simulink model "main"  (R2021a)
settings: Solver=ode113  StartTime=0.0  StopTime=100  RelTol=1e-13  AbsTol=1e-14
undefined symbols (not defined in the file or in its folder): Earth, initCond, Sensors, Spacecraft
libraries: aerolibutil x48, vrlib x31, dspsrcs4 x29, simulink x10, SADlibrary x8, commfilt2 x3, sharedtransform x3, dspfdesign x3, sharedutil x2, sharedTrackingLibrary x2, dspmathops x1
(part 1 of 3)
settings Model: Creator=matteo  LastModifiedBy=matteo
settings SolverCC: ZeroCrossControl=EnableAll  ZeroCrossAlgorithm=Adaptive  AlgebraicLoopSolver=TrustRegion  DecoupledContinuousIntegration=on
settings DebuggingCC: ReadBeforeWriteMsg=DisableAll  WriteAfterWriteMsg=DisableAll  WriteAfterReadMsg=DisableAll  MultiTaskDSMMsg=none  SFMachineParentedDataDiag=warning
settings ModelReferenceCC: UpdateModelReferenceTargets=IfOutOfDate
settings SFSimCC: SFSimEcho=off
settings SimscapeCC: SimscapeNormalizeSystem=off

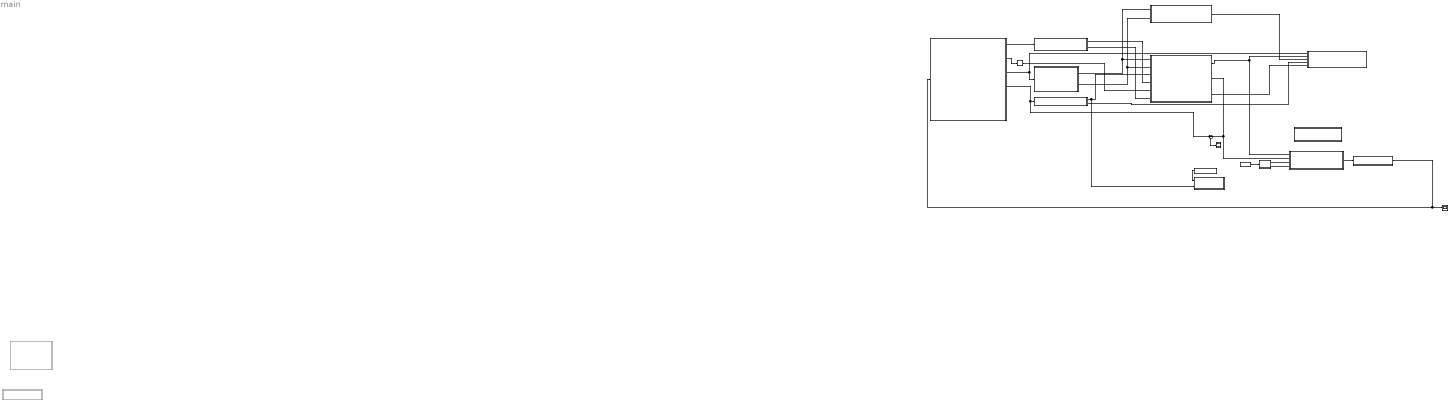
== system main ==
  Chart : Stateflow chart  Commented=on  TreatAsAtomicUnit=on
  Comparison : Subsystem
  Constant : Constant  Value=Spacecraft.str.inertia
  Control allocator : Subsystem
  Digital Clock : DigitalClock  SampleTime=1/1000
  Gyro reading : Subsystem
  Ideal control law : Subsystem
  Indipendent thrusters : Subsystem  Commented=on
  MATLAB Function : MATLAB Function  TreatAsAtomicUnit=on
  MATLAB Function4 : MATLAB Function  TreatAsAtomicUnit=on
  MPC : Subsystem
  Real physics : Subsystem
  Scope : Scope
  Scope4 : Scope
  Solve Whabba's problem : Subsystem
  Star sensor : Subsystem
  State estimator : Subsystem
  Subsystem1 : Subsystem
  Sum : Sum  Inputs=+-
  Zero-Order Hold : ZeroOrderHold  SampleTime=Sensors.sunSensor.freq
  wires:
  Real physics/4(Angular velocity [BF][rad/s]) -> Sum/1, Gyro reading/1(True ω [body refrence frame][rad/s])
  Real physics/2(Sun direction [NF]) -> Zero-Order Hold/1
  Real physics/1(Sun direction [BF]) -> Subsystem1/1(True Sun position [body reference frame][km])
  Real physics/3(q_B/N) -> Star sensor/1(Body attitude [Earth inertial frame]), Comparison/1(True attitude [ECI])
  Star sensor/1(Star 1 [SF]) -> Solve Whabba's problem/1(Stars [SF]), State estimator/1(Stars angles [sensor screen])
  Star sensor/2(in2) -> State estimator/2(MeasurementFcn1Inputs), Solve Whabba's problem/2(in2)
  Gyro reading/1(Measured ω [body reference frame][rad/s]) -> MATLAB Function4/2(omegaBody), State estimator/3(Gyro angular velocity [body frame])
  State estimator/1(Body frame attitude [ECI]) -> Comparison/2(Attitude Kalman [ECI]), Ideal control law/1(Body attitude [ECI])
  Solve Whabba's problem/1(Attitude quaternion) -> Comparison/3(Attitude Whabba's [ECI])
  State estimator/2(Angular velocity [body frame]) -> Sum/2, Ideal control law/2(Body angular speed [body frame])
  Gyro reading/2(Bias gyro true [body frame]) -> Comparison/4(Bias gyro true [body frame])
  State estimator/3(Gyro bias [body frame]) -> Comparison/5(Bias gyro Kalman [body frame])
  Sum/1 -> Scope/1
  MATLAB Function/1(q) -> Ideal control law/3(Reference attitude [ECI])
  MATLAB Function/2(omega) -> Ideal control law/4(Reference angular speed [ECI])
  Digital Clock/1 -> MATLAB Function/1(t)
  Control allocator/1(Real torque [body frame]) -> Real physics/1(Thrusters torque [BF][N m]), Scope4/1
  Subsystem1/1(Sun angles position [sensor axis]) -> State estimator/4(Sun sensor angles [SF])
  Zero-Order Hold/1 -> State estimator/5(Sun direction [NF])
  Subsystem1/2(Sensor attitude [body frame]) -> State estimator/6(Sun sensor attitude [BF])
  Constant/1 -> MATLAB Function4/1(J)
  Ideal control law/1(Ideal control torque [body frame]) -> Control allocator/1(Ideal torque [body frame])

== system main/Comparison ==
  True attitude [ECI] : Inport
  Attitude Kalman [ECI] : Inport  Port=2
  Attitude Whabba's [ECI] : Inport  Port=3
  Bias gyro true [body frame] : Inport  Port=4
  Bias gyro Kalman [body frame] : Inport  Port=5
  MATLAB Function : MATLAB Function  TreatAsAtomicUnit=on
  MATLAB Function1 : MATLAB Function  TreatAsAtomicUnit=on
  Quaternion Division1 : aerolibutil/Quaternion Division
      settings: SourceProductBaseCode=AE
  Quaternion Division2 : aerolibutil/Quaternion Division
      settings: SourceProductBaseCode=AE
  Scope : Scope  NumInputPorts=2
  Scope1 : Scope  NumInputPorts=2
  wires:
  True attitude [ECI]/1 -> Quaternion Division1/1, Quaternion Division2/1
  Attitude Kalman [ECI]/1 -> Quaternion Division2/2
  Attitude Whabba's [ECI]/1 -> Quaternion Division1/2
  Quaternion Division2/1 -> MATLAB Function1/1(q)  "UKF error"
  Bias gyro true [body frame]/1 -> Scope1/1
  Bias gyro Kalman [body frame]/1 -> Scope1/2
  MATLAB Function1/1(e) -> Scope/1  "UKF error"
  MATLAB Function/1(e) -> Scope/2  "Whabba's error"
  Quaternion Division1/1 -> MATLAB Function/1(q)  "Whabba's error"

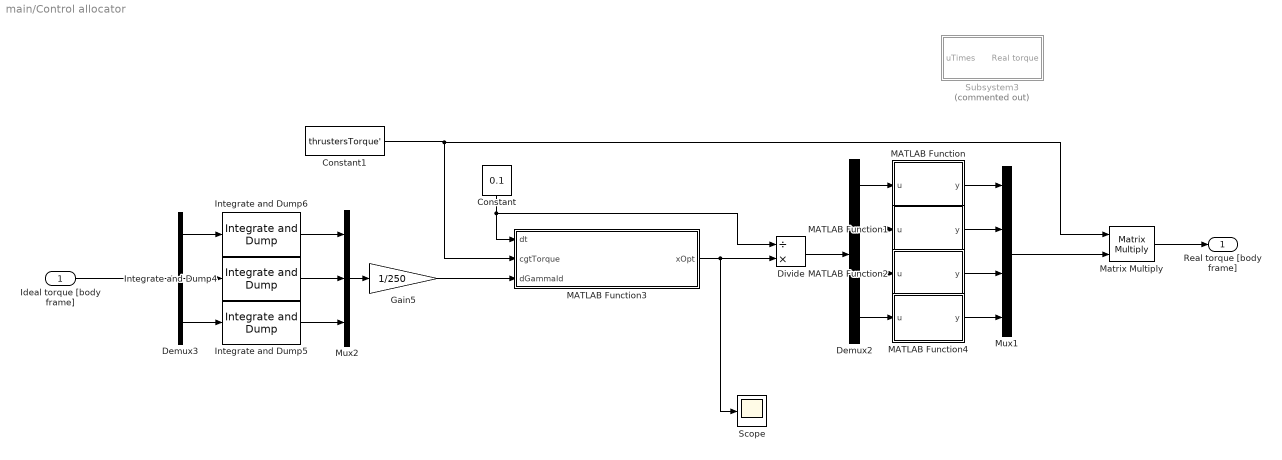
== system main/Control allocator ==
  Ideal torque [body frame] : Inport
  Constant : Constant  Value=0.1
  Constant1 : Constant  Value=thrustersTorque'  VectorParams1D=off
  Demux2 : Demux
  Demux3 : Demux  Outputs=3
  Divide : Product  Inputs=/*
  Gain5 : Gain  Gain=1/250
  Integrate and Dump4 : commfilt2/Integrate and Dump  obssamples=25  offsetsamples=0  nodump=off  roundingMode=Floor  overflowMode=off  outputDataTypeStr=Inherit: Same as accumulator  outputLastDataTypeStr=Inherit: Same as accumulator
  Integrate and Dump5 : commfilt2/Integrate and Dump  obssamples=25  offsetsamples=0  nodump=off  roundingMode=Floor  overflowMode=off  outputDataTypeStr=Inherit: Same as accumulator  outputLastDataTypeStr=Inherit: Same as accumulator
  Integrate and Dump6 : commfilt2/Integrate and Dump  obssamples=25  offsetsamples=0  nodump=off  roundingMode=Floor  overflowMode=off  outputDataTypeStr=Inherit: Same as accumulator  outputLastDataTypeStr=Inherit: Same as accumulator
  MATLAB Function : MATLAB Function  TreatAsAtomicUnit=on
  MATLAB Function1 : MATLAB Function  TreatAsAtomicUnit=on
  MATLAB Function2 : MATLAB Function  TreatAsAtomicUnit=on
  MATLAB Function3 : MATLAB Function  TreatAsAtomicUnit=on
  MATLAB Function4 : MATLAB Function  TreatAsAtomicUnit=on
  Matrix Multiply : Product  Multiplication=Matrix(*)
  Mux1 : Mux
  Mux2 : Mux  Inputs=3
  Scope : Scope
  Subsystem3 : Subsystem  Commented=on
  Real torque [body frame] : Outport
  wires:
  Integrate and Dump6/1 -> Mux2/1
  Demux3/2 -> Integrate and Dump4/1
  Gain5/1 -> MATLAB Function3/3(dGammaId)
  MATLAB Function3/1(xOpt) -> Divide/2, Scope/1
  Demux3/1 -> Integrate and Dump6/1
  Demux3/3 -> Integrate and Dump5/1
  Mux2/1 -> Gain5/1
  Integrate and Dump4/1 -> Mux2/2
  Ideal torque [body frame]/1 -> Demux3/1
  Integrate and Dump5/1 -> Mux2/3
  Constant/1 -> Divide/1, MATLAB Function3/1(dt)
  Demux2/4 -> MATLAB Function4/1(u)
  Mux1/1 -> Matrix Multiply/2
  MATLAB Function4/1(y) -> Mux1/4
  Matrix Multiply/1 -> Real torque [body frame]/1
  Demux2/3 -> MATLAB Function2/1(u)
  MATLAB Function/1(y) -> Mux1/1
  Demux2/1 -> MATLAB Function/1(u)
  MATLAB Function2/1(y) -> Mux1/3
  Constant1/1 -> MATLAB Function3/2(cgtTorque), Matrix Multiply/1
  Divide/1 -> Demux2/1
  MATLAB Function1/1(y) -> Mux1/2
  Demux2/2 -> MATLAB Function1/1(u)

== system main/Gyro reading ==
  True ω [body refrence frame][rad/s] : Inport
  Constant : Constant  Value=1e-3*randn(3,1)
  Cumulative Sum : dspmathops/Cumulative Sum  dim=Channels (running sum)  reset_popup=None  roundingMode=Floor  overflowMode=off  outputDataTypeStr=Inherit: Same as accumulator  outputMin=[]  outputMax=[]  outputLastDataTypeStr=Inherit: Same as accumulator
  Gain : Gain  Gain=sqrt(1/Sensors.gyro.freq)
  Random Source : dspsrcs4/Random Source  SrcType=Gaussian  NormMethod=Ziggurat  CltLength=12  MinVal=0  MaxVal=1  MeanVal=0  VarVal=Sensors.gyro.acc  RepMode=Not repeatable  rawSeed=1  IsInherit=off  SampMode=Discrete  SampTime=1/Sensors.gyro.freq  SampFrame=3  DataType=Double  OutComplex=Real  OutputFrames=off
  Random Source1 : dspsrcs4/Random Source  SrcType=Gaussian  NormMethod=Ziggurat  CltLength=12  MinVal=0  MaxVal=1  MeanVal=0  VarVal=Sensors.gyro.biasInstability  RepMode=Not repeatable  rawSeed=1  IsInherit=off  SampMode=Discrete  SampTime=1/Sensors.gyro.freq  SampFrame=3  DataType=Double  OutComplex=Real  OutputFrames=off
  Sum : Sum  Inputs=|++
  Sum1 : Sum  Inputs=|++
  Sum2 : Sum  Inputs=|++
  Zero-Order Hold : ZeroOrderHold  SampleTime=1/Sensors.gyro.freq
  Measured ω [body reference frame][rad/s] : Outport
  Bias gyro true [body frame] : Outport  Port=2
  wires:
  Sum2/1 -> Measured ω [body reference frame][rad/s]/1
  True ω [body refrence frame][rad/s]/1 -> Zero-Order Hold/1
  Cumulative Sum/1 -> Sum1/2
  Gain/1 -> Cumulative Sum/1
  Random Source1/1 -> Gain/1
  Constant/1 -> Sum1/1
  Zero-Order Hold/1 -> Sum/1
  Random Source/1 -> Sum/2
  Sum/1 -> Sum2/1
  Sum1/1 -> Bias gyro true [body frame]/1, Sum2/2

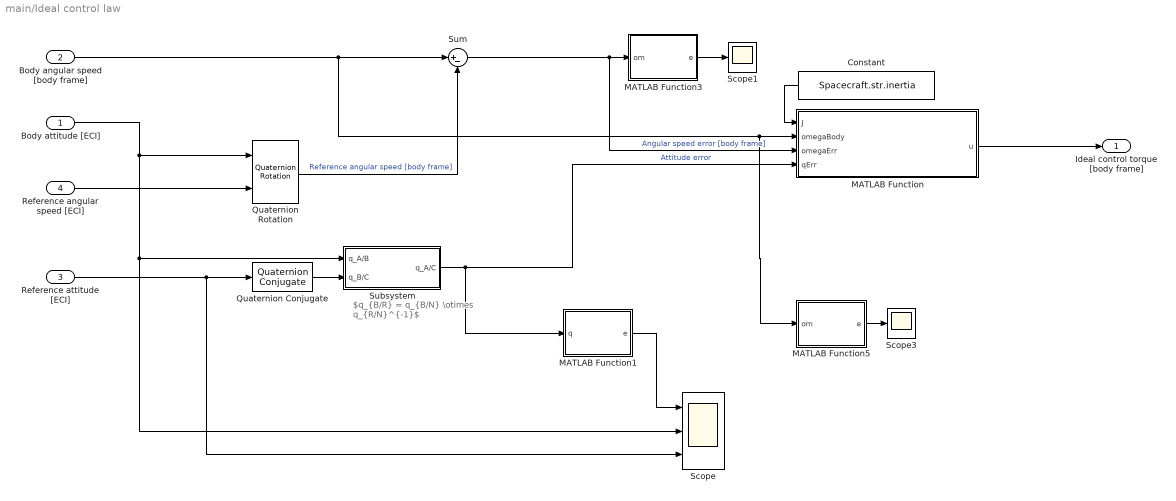
== system main/Ideal control law ==
  note: $q_{B/R} = q_{B/N} \otimes q_{R/N}^{-1}$
  Body attitude [ECI] : Inport
  Body angular speed [body frame] : Inport  Port=2
  Reference attitude [ECI] : Inport  Port=3
  Reference angular speed [ECI] : Inport  Port=4
  Constant : Constant  Value=Spacecraft.str.inertia
  MATLAB Function : MATLAB Function  TreatAsAtomicUnit=on
  MATLAB Function1 : MATLAB Function  TreatAsAtomicUnit=on
  MATLAB Function3 : MATLAB Function  TreatAsAtomicUnit=on
  MATLAB Function5 : MATLAB Function  TreatAsAtomicUnit=on
  Quaternion Conjugate : aerolibutil/Quaternion Conjugate
      settings: SourceProductBaseCode=AE
  Quaternion Rotation : aerolibutil/Quaternion Rotation
  Scope : Scope  NumInputPorts=3
  Scope1 : Scope
  Scope3 : Scope
  Subsystem : Subsystem
  Sum : Sum  Inputs=|+-
  Ideal control torque [body frame] : Outport
  wires:
  Subsystem/1(q_A/C) -> MATLAB Function/4(qErr), MATLAB Function1/1(q)  "Attitude error"
  Reference angular speed [ECI]/1 -> Quaternion Rotation/2
  Quaternion Rotation/1 -> Sum/2  "Reference angular speed [body frame]"
  Body angular speed [body frame]/1 -> MATLAB Function5/1(om), MATLAB Function/2(omegaBody), Sum/1
  Sum/1 -> MATLAB Function3/1(om), MATLAB Function/3(omegaErr)  "Angular speed error [body frame]"
  Constant/1 -> MATLAB Function/1(J)
  Reference attitude [ECI]/1 -> Scope/3, Quaternion Conjugate/1
  Body attitude [ECI]/1 -> Scope/2, Subsystem/1(q_A/B), Quaternion Rotation/1
  MATLAB Function1/1(e) -> Scope/1
  MATLAB Function3/1(e) -> Scope1/1
  MATLAB Function5/1(e) -> Scope3/1
  MATLAB Function/1(u) -> Ideal control torque [body frame]/1
  Quaternion Conjugate/1 -> Subsystem/2(q_B/C)

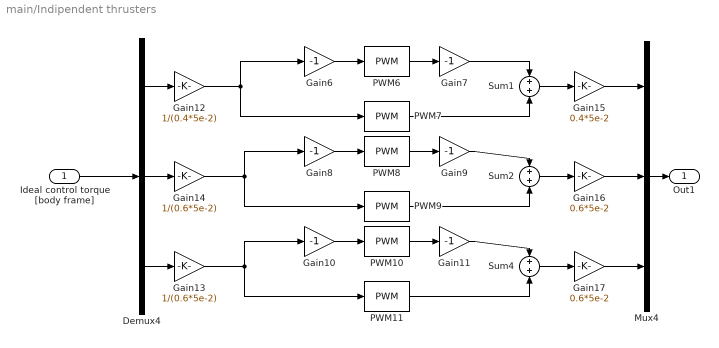
== system main/Indipendent thrusters ==
  Ideal control torque [body frame] : Inport
  Demux4 : Demux  Outputs=3
  Gain{6..11} (6 alike) : Gain  Gain=-1
  Gain12 : Gain  Gain=1/(0.4*5e-2)
  Gain13 : Gain  Gain=1/(0.6*5e-2)
  Gain14 : Gain  Gain=1/(0.6*5e-2)
  Gain15 : Gain  Gain=0.4*5e-2
  Gain16 : Gain  Gain=0.6*5e-2
  Gain17 : Gain  Gain=0.6*5e-2
  Mux4 : Mux  Inputs=3
  PWM{6..11} (6 alike) : simulink/Discontinuities/PWM  DisableCoverage=on  Period=0.5  DisallowZeroDutyCycle=off  RunAtFixedTimeIntervals=on  SampleTime=1/Sensors.gyroSamplingFreq
  Sum1 : Sum
  Sum2 : Sum
  Sum4 : Sum
  Out1 : Outport
  wires:
  PWM8/1 -> Gain9/1
  Mux4/1 -> Out1/1
  PWM11/1 -> Sum4/2
  Gain11/1 -> Sum4/1
  PWM6/1 -> Gain7/1
  Sum2/1 -> Gain16/1
  PWM10/1 -> Gain11/1
  Gain12/1 -> PWM7/1, Gain6/1
  Gain17/1 -> Mux4/3
  PWM7/1 -> Sum1/2
  Gain6/1 -> PWM6/1
  Gain16/1 -> Mux4/2
  Gain9/1 -> Sum2/1
  Gain14/1 -> PWM9/1, Gain8/1
  Demux4/1 -> Gain12/1
  Gain10/1 -> PWM10/1
  Gain13/1 -> PWM11/1, Gain10/1
  Demux4/2 -> Gain14/1
  Sum4/1 -> Gain17/1
  Ideal control torque [body frame]/1 -> Demux4/1
  Sum1/1 -> Gain15/1
  Gain8/1 -> PWM8/1
  Gain15/1 -> Mux4/1
  Demux4/3 -> Gain13/1
  PWM9/1 -> Sum2/2
  Gain7/1 -> Sum1/1

== system main/MPC ==
  Body attitude [ECI] : Inport
  Body angular speed [BF] : Inport  Port=2
  MATLAB Function : MATLAB Function  TreatAsAtomicUnit=on
  Ideal control law [BF] : Outport

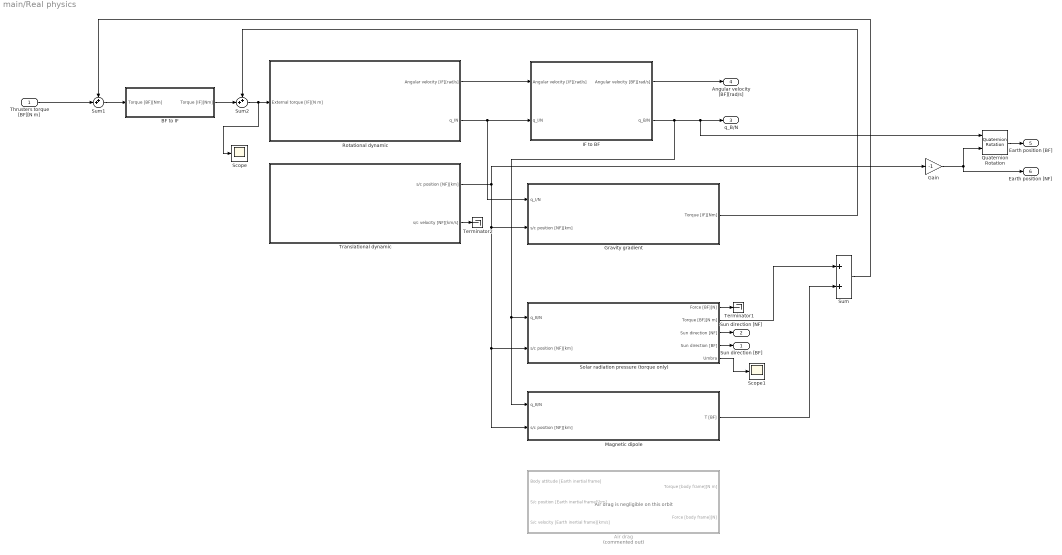
== system main/Real physics ==
  note: Air drag is negligible on this orbit
  Thrusters torque [BF][N m] : Inport  Unit=N*m
  Air drag : Subsystem  Commented=on
  BF to IF : Subsystem
  Gain : Gain  Gain=-1
  Gravity gradient : Subsystem
  IF to BF : Subsystem
  Magnetic dipole : Subsystem
  Quaternion Rotation : aerolibutil/Quaternion Rotation
  Rotational dynamic : Subsystem
  Scope : Scope
  Scope1 : Scope
  Solar radiation pressure (torque only) : Subsystem
  Sum : Sum
  Sum1 : Sum  Inputs=++|
  Sum2 : Sum  Inputs=++|
  Terminator1 : Terminator
  Terminator2 : Terminator
  Translational dynamic : Subsystem
  Sun direction [BF] : Outport  OutDataTypeStr=double  Unit=km
  Sun direction [NF] : Outport  Port=2
  q_B/N : Outport  Port=3
  Angular velocity [BF][rad/s] : Outport  Port=4
  Earth position [BF] : Outport  Port=5
  Earth position [NF] : Outport  Port=6
  wires:
  Sum/1 -> Sum1/1
  Solar radiation pressure (torque only)/1(Force [BF][N]) -> Terminator1/1
  Solar radiation pressure (torque only)/2(Torque [BF][N m]) -> Sum/1
  Thrusters torque [BF][N m]/1 -> Sum1/2
  Sum1/1 -> BF to IF/1(Torque [BF][Nm])
  Translational dynamic/1(s/c position [NF][km]) -> Solar radiation pressure (torque only)/2(s/c position [NF][km]), Magnetic dipole/2(s/c position [NF][km]), Gravity gradient/2(s/c position [NF][km]), Gain/1
  Rotational dynamic/1(Angular velocity [IF][rad/s]) -> IF to BF/1(Angular velocity [IF][rad/s])
  IF to BF/1(Angular velocity [BF][rad/s]) -> Angular velocity [BF][rad/s]/1
  IF to BF/2(q_B/N) -> Magnetic dipole/1(q_B/N), Solar radiation pressure (torque only)/1(q_B/N), q_B/N/1, Quaternion Rotation/1
  Solar radiation pressure (torque only)/3(Sun direction [NF]) -> Sun direction [NF]/1
  Solar radiation pressure (torque only)/4(Sun direction [BF]) -> Sun direction [BF]/1
  Solar radiation pressure (torque only)/5(Umbra) -> Scope1/1
  BF to IF/1(Torque [IF][Nm]) -> Sum2/2
  Sum2/1 -> Scope/1, Rotational dynamic/1(External torque [IF][N m])
  Translational dynamic/2(s/c velocity [NF][km/s]) -> Terminator2/1
  Gravity gradient/1(Torque [IF][Nm]) -> Sum2/1
  Rotational dynamic/2(q_IN) -> Gravity gradient/1(q_I/N), IF to BF/2(q_I/N)
  Gain/1 -> Earth position [NF]/1, Quaternion Rotation/2
  Quaternion Rotation/1 -> Earth position [BF]/1
  Magnetic dipole/1(T [BF]) -> Sum/2

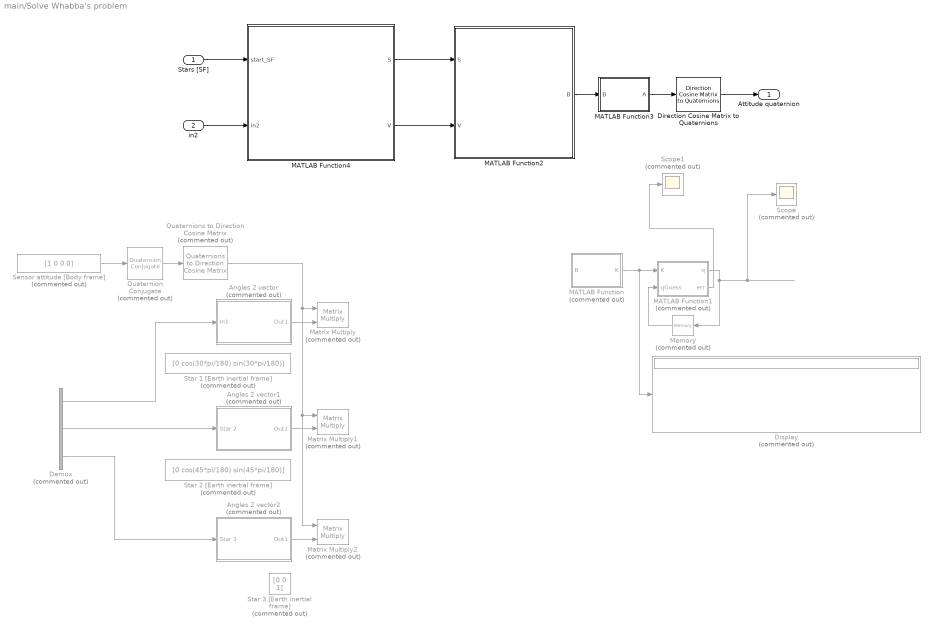
== system main/Solve Whabba's problem ==
  Stars [SF] : Inport
  in2 : Inport  Port=2
  Angles 2 vector : Subsystem  Commented=on
  Angles 2 vector1 : Subsystem  Commented=on
  Angles 2 vector2 : Subsystem  Commented=on
  Demux : Demux  Commented=on  Outputs=3
  Direction Cosine Matrix to Quaternions : sharedtransform/Direction Cosine Matrix  to Quaternions  aMode=0  action=None  tolerance=eps(2)
      settings: SourceProductBaseCode=AE,PW,DR,MT,UV,VE
  Display : Display  Commented=on
  MATLAB Function : MATLAB Function  Commented=on  TreatAsAtomicUnit=on
  MATLAB Function1 : MATLAB Function  Commented=on  TreatAsAtomicUnit=on
  MATLAB Function2 : MATLAB Function  TreatAsAtomicUnit=on
  MATLAB Function3 : MATLAB Function  TreatAsAtomicUnit=on
  MATLAB Function4 : MATLAB Function  TreatAsAtomicUnit=on
  Matrix Multiply : Product  Commented=on  Multiplication=Matrix(*)
  Matrix Multiply1 : Product  Commented=on  Multiplication=Matrix(*)
  Matrix Multiply2 : Product  Commented=on  Multiplication=Matrix(*)
  Memory : Memory  Commented=on  InitialCondition=[1 0 0 0]
  Quaternion Conjugate : aerolibutil/Quaternion Conjugate  Commented=on
      settings: SourceProductBaseCode=AE
  Quaternions to Direction Cosine Matrix : sharedtransform/Quaternions to  Direction Cosine Matrix  Commented=on  aMode=aMode
      settings: SourceProductBaseCode=AE,PW,DR,MT,UV,VE
  Scope : Scope  Commented=on
  Scope1 : Scope  Commented=on
  Sensor attitude [Body frame] : Constant  Commented=on  Value=[1 0 0 0]
  Star 1 [Earth inertial frame] : Constant  Commented=on  Value=[0 cos(30*pi/180) sin(30*pi/180)]
  Star 2 [Earth inertial frame] : Constant  Commented=on  Value=[0 cos(45*pi/180) sin(45*pi/180)]
  Star 3 [Earth inertial frame] : Constant  Commented=on  Value=[0 0 1]
  Attitude quaternion : Outport
  wires:
  Demux/1 -> Angles 2 vector/1(In1)
  Demux/2 -> Angles 2 vector1/1(Star 2)
  Demux/3 -> Angles 2 vector2/1(Star 3)
  Angles 2 vector/1(Out1) -> Matrix Multiply/2
  MATLAB Function2/1(B) -> MATLAB Function3/1(B)
  MATLAB Function/1(K) -> Display/1, MATLAB Function1/1(K)
  MATLAB Function1/1(q) -> Memory/1, Scope/1
  Sensor attitude [Body frame]/1 -> Quaternion Conjugate/1
  Quaternion Conjugate/1 -> Quaternions to Direction Cosine Matrix/1
  Quaternions to Direction Cosine Matrix/1 -> Matrix Multiply2/1, Matrix Multiply1/1, Matrix Multiply/1
  Angles 2 vector2/1(Out1) -> Matrix Multiply2/2
  Angles 2 vector1/1(Out1) -> Matrix Multiply1/2
  Memory/1 -> MATLAB Function1/2(qGuess)
  MATLAB Function1/2(err) -> Scope1/1
  MATLAB Function3/1(A) -> Direction Cosine Matrix to Quaternions/1
  Direction Cosine Matrix to Quaternions/1 -> Attitude quaternion/1
  MATLAB Function4/1(S) -> MATLAB Function2/1(S)
  MATLAB Function4/2(V) -> MATLAB Function2/2(V)
  Stars [SF]/1 -> MATLAB Function4/1(start_SF)
  in2/1 -> MATLAB Function4/2(in2)

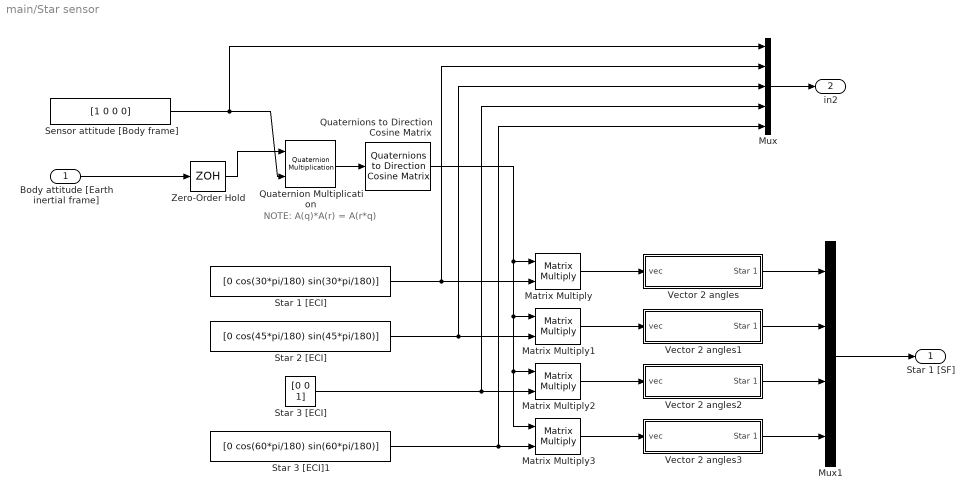
== system main/Star sensor ==
  note: NOTE: A(q)*A(r) = A(r*q)
  Body attitude [Earth inertial frame] : Inport
  Matrix Multiply{,1..3} (4 alike) : Product  Multiplication=Matrix(*)
  Mux : Mux  Inputs=5
  Mux1 : Mux
  Quaternion Multiplication : aerolibutil/Quaternion Multiplication
  Quaternions to Direction Cosine Matrix : sharedtransform/Quaternions to  Direction Cosine Matrix  aMode=aMode
      settings: SourceProductBaseCode=AE,PW,DR,MT,UV,VE
  Sensor attitude [Body frame] : Constant  Value=[1 0 0 0]
  Star 1 [ECI] : Constant  Value=[0 cos(30*pi/180) sin(30*pi/180)]
  Star 2 [ECI] : Constant  Value=[0 cos(45*pi/180) sin(45*pi/180)]
  Star 3 [ECI] : Constant  Value=[0 0 1]
  Star 3 [ECI]1 : Constant  Value=[0 cos(60*pi/180) sin(60*pi/180)]
  Vector 2 angles : Subsystem
  Vector 2 angles1 : Subsystem
  Vector 2 angles2 : Subsystem
  Vector 2 angles3 : Subsystem
  Zero-Order Hold : ZeroOrderHold  SampleTime=1/Sensors.starTracker.freq
  Star 1 [SF] : Outport
  in2 : Outport  Port=2
  wires:
  Body attitude [Earth inertial frame]/1 -> Zero-Order Hold/1
  Sensor attitude [Body frame]/1 -> Quaternion Multiplication/2, Mux/1
  Quaternion Multiplication/1 -> Quaternions to Direction Cosine Matrix/1
  Star 1 [ECI]/1 -> Matrix Multiply/2, Mux/2
  Star 2 [ECI]/1 -> Mux/3, Matrix Multiply1/2
  Star 3 [ECI]/1 -> Mux/4, Matrix Multiply2/2
  Quaternions to Direction Cosine Matrix/1 -> Matrix Multiply3/1, Matrix Multiply2/1, Matrix Multiply1/1, Matrix Multiply/1
  Matrix Multiply/1 -> Vector 2 angles/1(vec)
  Matrix Multiply2/1 -> Vector 2 angles2/1(vec)
  Matrix Multiply1/1 -> Vector 2 angles1/1(vec)
  Vector 2 angles1/1(Star 1) -> Mux1/2
  Vector 2 angles2/1(Star 1) -> Mux1/3
  Vector 2 angles/1(Star 1) -> Mux1/1
  Mux/1 -> in2/1
  Zero-Order Hold/1 -> Quaternion Multiplication/1
  Mux1/1 -> Star 1 [SF]/1
  Star 3 [ECI]1/1 -> Mux/5, Matrix Multiply3/2
  Matrix Multiply3/1 -> Vector 2 angles3/1(vec)
  Vector 2 angles3/1(Star 1) -> Mux1/4

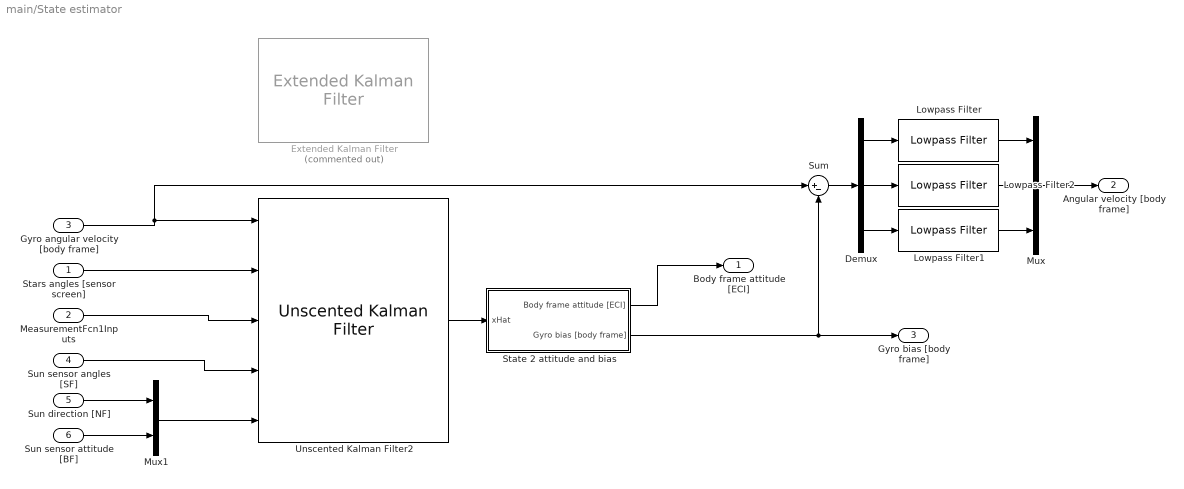
== system main/State estimator ==
  Stars angles [sensor screen] : Inport
  MeasurementFcn1Inputs : Inport  Port=2
  Gyro angular velocity [body frame] : Inport  Port=3
  Sun sensor angles [SF] : Inport  Port=4
  Sun direction [NF] : Inport  Port=5
  Sun sensor attitude [BF] : Inport  Port=6
  Demux : Demux  Outputs=3
  Extended Kalman Filter : sharedTrackingLibrary/Extended Kalman Filter  Commented=on  StateTransitionFcn=statePropagation  HasStateTransitionJacobianFcn=off  HasAdditiveProcessNoise=Nonadditive  ProcessNoise=diag([Sensors.gyro.acc* [1 1 1], Sensors.gyro.biasInstability* [1 1 1]])  HasTimeVaryingProcessNoise=off  HasStateTransitionFcnExtraArgument=1  InitialState=[Spacecraft.initialAttitude 0 0 0]'  InitialStateCovariance=1e-6*eye(7)  MeasurementFcn1=simulateStarTracker  HasMeasurementJacobianFcn1=off  HasMeasurementEnablePort1=off  HasAdditiveMeasurementNoise1=Additive  MeasurementNoise1=diag(repmat([Sensors.sunSensor.aboutBoresight Sensors.sunSensor.crossBoresight Sensors.sunSensor.crossBoresight],[1 4]));  HasTimeVaryingMeasurementNoise1=off  HasMeasurementFcnExtraArgument1=1  MeasurementFcn2=simulateSunSensor  HasMeasurementJacobianFcn2=off  HasMeasurementEnablePort2=off  HasAdditiveMeasurementNoise2=Additive  MeasurementNoise2=diag([Sensors.sunSensor.aboutBoresight Sensors.sunSensor.crossBoresight Sensors.sunSensor.crossBoresight]);  HasTimeVaryingMeasurementNoise2=off  HasMeasurementFcnExtraArgument2=1  MeasurementFcn3=myMeasurementFcn  HasMeasurementJacobianFcn3=off  HasMeasurementEnablePort3=off  HasAdditiveMeasurementNoise3=Additive  MeasurementNoise3=1  HasTimeVaryingMeasurementNoise3=off  HasMeasurementFcnExtraArgument3=0  MeasurementFcn4=myMeasurementFcn  HasMeasurementJacobianFcn4=off  HasMeasurementEnablePort4=off  HasAdditiveMeasurementNoise4=Additive  MeasurementNoise4=1  HasTimeVaryingMeasurementNoise4=off  HasMeasurementFcnExtraArgument4=0  MeasurementFcn5=myMeasurementFcn  HasMeasurementJacobianFcn5=off  HasMeasurementEnablePort5=off  HasAdditiveMeasurementNoise5=Additive  MeasurementNoise5=1  HasTimeVaryingMeasurementNoise5=off  HasMeasurementFcnExtraArgument5=0  EnableMultirate=on  StateTransitionFcnSampleTime=1/Sensors.gyro.freq  MeasurementFcn1SampleTime=1/Sensors.starTracker.freq  MeasurementFcn2SampleTime=1/Sensors.sunSensor.freq  MeasurementFcn3SampleTime=1  MeasurementFcn4SampleTime=1  MeasurementFcn5SampleTime=1  UseCurrentEstimator=on  OutputStateCovariance=off  DataType=double  SampleTime=1  NumberOfMeasurements=2
      settings: SourceProductBaseCode=CT,DR,TF,ID,LP,NV,AR,RO,RR,UV,VE
  Lowpass Filter : dspfdesign/Lowpass Filter  FilterType=FIR  DesignForMinimumOrder=on  FilterOrder=50  PassbandFrequency=20  StopbandFrequency=40  PassbandRipple=0.0001  StopbandAttenuation=80  InheritSampleRate=off  SampleRate=250  SimulateUsing=Interpreted execution  roundingMode=Floor  coeffsDataTypeStr=fixdt(1,16)
  Lowpass Filter1 : dspfdesign/Lowpass Filter  FilterType=FIR  DesignForMinimumOrder=on  FilterOrder=50  PassbandFrequency=20  StopbandFrequency=40  PassbandRipple=0.0001  StopbandAttenuation=80  InheritSampleRate=off  SampleRate=250  SimulateUsing=Interpreted execution  roundingMode=Floor  coeffsDataTypeStr=fixdt(1,16)
  Lowpass Filter2 : dspfdesign/Lowpass Filter  FilterType=FIR  DesignForMinimumOrder=on  FilterOrder=50  PassbandFrequency=20  StopbandFrequency=40  PassbandRipple=0.0001  StopbandAttenuation=80  InheritSampleRate=off  SampleRate=250  SimulateUsing=Interpreted execution  roundingMode=Floor  coeffsDataTypeStr=fixdt(1,16)
  Mux : Mux  Inputs=3
  Mux1 : Mux  Inputs=2
  State 2 attitude and bias : Subsystem
  Sum : Sum  Inputs=|+-
  Unscented Kalman Filter2 : sharedTrackingLibrary/Unscented Kalman Filter  StateTransitionFcn=statePropagation  HasAdditiveProcessNoise=Nonadditive  ProcessNoise=diag([Sensors.gyro.acc* [1 1 1], Sensors.gyro.biasInstability * [1 1 1]])  HasTimeVaryingProcessNoise=off  HasStateTransitionFcnExtraArgument=1  InitialState=[Spacecraft.initialAttitude 0 0 0]'  InitialStateCovariance=1e-6*eye(7)  Alpha=1e-3  Beta=2  Kappa=0  MeasurementFcn1=simulateStarTracker  HasMeasurementEnablePort1=off  HasAdditiveMeasurementNoise1=Nonadditive  MeasurementNoise1=diag(repmat([Sensors.starTracker.aboutBoresight Sensors.starTracker.crossBoresight],[1 4]));  HasTimeVaryingMeasurementNoise1=off  HasMeasurementFcnExtraArgument1=1  MeasurementFcn2=simulateSunSensor  HasMeasurementEnablePort2=off  HasAdditiveMeasurementNoise2=Nonadditive  MeasurementNoise2=diag([Sensors.sunSensor.aboutBoresight Sensors.sunSensor.crossBoresight]);  HasTimeVaryingMeasurementNoise2=off  HasMeasurementFcnExtraArgument2=1  MeasurementFcn3=simulateSunSensor  HasMeasurementEnablePort3=off  HasAdditiveMeasurementNoise3=Additive  MeasurementNoise3=(.1*pi/180)^2*eye(2)  HasTimeVaryingMeasurementNoise3=off  HasMeasurementFcnExtraArgument3=1  MeasurementFcn4=myMeasurementFcn  HasMeasurementEnablePort4=off  HasAdditiveMeasurementNoise4=Additive  MeasurementNoise4=1  HasTimeVaryingMeasurementNoise4=off  HasMeasurementFcnExtraArgument4=0  MeasurementFcn5=myMeasurementFcn  HasMeasurementEnablePort5=off  HasAdditiveMeasurementNoise5=Additive  MeasurementNoise5=1  HasTimeVaryingMeasurementNoise5=off  HasMeasurementFcnExtraArgument5=0  EnableMultirate=on  StateTransitionFcnSampleTime=1/Sensors.gyro.freq  MeasurementFcn1SampleTime=1/Sensors.starTracker.freq  MeasurementFcn2SampleTime=1/Sensors.sunSensor.freq  MeasurementFcn3SampleTime=Sensors.sunSensorSamplingFreq  MeasurementFcn4SampleTime=1  MeasurementFcn5SampleTime=1  UseCurrentEstimator=on  OutputStateCovariance=off  DataType=double  SampleTime=0.01  NumberOfMeasurements=2
      settings: SourceProductBaseCode=CT,DR,TF,ID,LP,NV,AR,RO,RR,UV,VE
  Body frame attitude [ECI] : Outport
  Angular velocity [body frame] : Outport  Port=2
  Gyro bias [body frame] : Outport  Port=3
  wires:
  MeasurementFcn1Inputs/1 -> Unscented Kalman Filter2/3
  State 2 attitude and bias/2(Gyro bias [body frame]) -> Sum/2, Gyro bias [body frame]/1
  State 2 attitude and bias/1(Body frame attitude [ECI]) -> Body frame attitude [ECI]/1
  Unscented Kalman Filter2/1 -> State 2 attitude and bias/1(xHat)
  Stars angles [sensor screen]/1 -> Unscented Kalman Filter2/2
  Demux/1 -> Lowpass Filter/1
  Demux/2 -> Lowpass Filter2/1
  Demux/3 -> Lowpass Filter1/1
  Lowpass Filter/1 -> Mux/1
  Lowpass Filter1/1 -> Mux/3
  Lowpass Filter2/1 -> Mux/2
  Sum/1 -> Demux/1
  Mux/1 -> Angular velocity [body frame]/1
  Gyro angular velocity [body frame]/1 -> Unscented Kalman Filter2/1, Sum/1
  Sun sensor angles [SF]/1 -> Unscented Kalman Filter2/4
  Mux1/1 -> Unscented Kalman Filter2/5
  Sun direction [NF]/1 -> Mux1/1
  Sun sensor attitude [BF]/1 -> Mux1/2

== system main/Subsystem1 ==
  True Sun position [body reference frame][km] : Inport
  MATLAB Function1 : MATLAB Function  TreatAsAtomicUnit=on
  Sensor orientation : Constant  Value=[1 0 0 0]
  Sensor orientation1 : Constant  Value=[cos(pi/4) 0 sin(pi/4) 0]
  Sensor orientation2 : Constant  Value=[cos(pi/2) 0 sin(pi/2) 0]
  Sensor orientation3 : Constant  Value=[cos(pi/4) 0 -sin(pi/4) 0]
  Sensor orientation4 : Constant  Value=[cos(pi/4) -sin(pi/4) 0 0]
  Sensor orientation5 : Constant  Value=[cos(pi/4) sin(pi/4) 0 0]
  Sun sensor reading : Subsystem
  Sun sensor reading1 : Subsystem
  Sun sensor reading2 : Subsystem
  Sun sensor reading3 : Subsystem
  Sun sensor reading4 : Subsystem
  Sun sensor reading5 : Subsystem
  Sun angles position [sensor axis] : Outport  PortDimensions=2
  Sensor attitude [body frame] : Outport  Port=2  PortDimensions=4
  wires:
  True Sun position [body reference frame][km]/1 -> Sun sensor reading2/1(True Sun position [body reference frame][km]), Sun sensor reading1/1(True Sun position [body reference frame][km]), Sun sensor reading/1(True Sun position [body reference frame][km]), Sun sensor reading3/1(True Sun position [body reference frame][km]), Sun sensor reading5/1(True Sun position [body reference frame][km]), Sun sensor reading4/1(True Sun position [body reference frame][km])
  MATLAB Function1/2(sensAtt) -> Sensor attitude [body frame]/1
  Sun sensor reading/1(Sun angles position [sensor axis]) -> MATLAB Function1/1(s1)
  MATLAB Function1/1(s) -> Sun angles position [sensor axis]/1
  Sensor orientation/1 -> MATLAB Function1/2(q_SB1), Sun sensor reading/2(q_S/B)
  Sun sensor reading1/1(Sun angles position [sensor axis]) -> MATLAB Function1/3(s2)
  Sun sensor reading2/1(Sun angles position [sensor axis]) -> MATLAB Function1/5(s3)
  Sun sensor reading3/1(Sun angles position [sensor axis]) -> MATLAB Function1/7(s4)
  Sun sensor reading4/1(Sun angles position [sensor axis]) -> MATLAB Function1/9(s5)
  Sun sensor reading5/1(Sun angles position [sensor axis]) -> MATLAB Function1/11(s6)
  Sensor orientation1/1 -> Sun sensor reading1/2(q_S/B), MATLAB Function1/4(q_SB2)
  Sensor orientation2/1 -> Sun sensor reading2/2(q_S/B), MATLAB Function1/6(q_SB3)
  Sensor orientation3/1 -> Sun sensor reading3/2(q_S/B), MATLAB Function1/8(q_SB4)
  Sensor orientation4/1 -> Sun sensor reading4/2(q_S/B), MATLAB Function1/10(q_SB5)
  Sensor orientation5/1 -> Sun sensor reading5/2(q_S/B), MATLAB Function1/12(q_SB6)

== system main/Control allocator/Subsystem3 ==
  uTimes : Inport
  Constant : Constant  Value=thrustersTorque'  VectorParams1D=off
  Demux1 : Demux  Commented=on
  Demux2 : Demux
  Gain : Gain  Gain=1/(50/500)
  MATLAB Function : MATLAB Function  TreatAsAtomicUnit=on
  MATLAB Function1 : MATLAB Function  TreatAsAtomicUnit=on
  MATLAB Function2 : MATLAB Function  TreatAsAtomicUnit=on
  MATLAB Function3 : MATLAB Function  TreatAsAtomicUnit=on
  Matrix Multiply : Product  Multiplication=Matrix(*)
  Mux1 : Mux  Commented=on
  Mux2 : Mux
  PWM{13,17..18,21} (4 alike) : simulink/Discontinuities/PWM  Commented=on  DisableCoverage=on  Period=0.1  DisallowZeroDutyCycle=off  RunAtFixedTimeIntervals=on  SampleTime=0.1
  Real torque : Outport
  wires:
  Mux2/1 -> Matrix Multiply/2
  Constant/1 -> Matrix Multiply/1
  Matrix Multiply/1 -> ?
  PWM18/1 -> Mux1/3
  PWM21/1 -> Mux1/1
  Demux1/2 -> PWM17/1
  PWM17/1 -> Mux1/2
  PWM13/1 -> Mux1/4
  Demux1/1 -> PWM21/1
  Demux1/4 -> PWM13/1
  Demux1/3 -> PWM18/1
  uTimes/1 -> ?
  Demux2/1 -> MATLAB Function/1(u)
  Gain/1 -> Demux2/1
  MATLAB Function/1(y) -> Mux2/1
  Demux2/2 -> MATLAB Function1/1(u)
  MATLAB Function1/1(y) -> Mux2/2
  Demux2/3 -> MATLAB Function2/1(u)
  MATLAB Function2/1(y) -> Mux2/3
  Demux2/4 -> MATLAB Function3/1(u)
  MATLAB Function3/1(y) -> Mux2/4

== system main/Ideal control law/Subsystem ==
  q_A/B : Inport
  q_B/C : Inport  Port=2
  Quaternion Multiplication : aerolibutil/Quaternion Multiplication
  q_A/C : Outport
  wires:
  q_A/B/1 -> Quaternion Multiplication/2
  q_B/C/1 -> Quaternion Multiplication/1
  Quaternion Multiplication/1 -> q_A/C/1

== system main/Real physics/Air drag ==
  Body attitude [Earth inertial frame] : Inport  Unit=1
  S/c position [Earth inertial frame][km] : Inport  Port=2  OutDataTypeStr=double  Unit=km  PortDimensions=3
  S/c velocity [Earth inertial frame][km/s] : Inport  Port=3  OutDataTypeStr=double  Unit=km/s
  Air density : Subsystem
  Constant : Constant  Value=Spacecraft  OutDataTypeStr=Bus: SpacecraftDT
  Constant1 : Constant  Value=Earth.equatorialRadius
  Constant2 : Constant  Value=2*pi/Earth.siderealDay
  Cross Product : vrlib/Utilities/Cross Product
  Gain : Gain  Gain=[0;0;1]
  MATLAB Function : MATLAB Function  TreatAsAtomicUnit=on
  Sum : Sum  Inputs=+-|
  Sum1 : Sum  Inputs=|-+
  Terminator : Terminator
  Vector magnitude and direction1 : SADlibrary/Vector magnitude and direction  SystemSampleTime=-1  VariantActivationTime=update diagram  Latency=0  AutoFrameSizeCalculation=off
  Vector rotate : SADlibrary/Vector rotate  SystemSampleTime=-1  VariantActivationTime=update diagram  Latency=0  AutoFrameSizeCalculation=off
  Torque [body frame][N m] : Outport  Unit=N*m
  Force [body frame][N] : Outport  Port=2  Unit=N
  wires:
  Vector magnitude and direction1/1 -> Sum/1
  Body attitude [Earth inertial frame]/1 -> Vector rotate/1
  MATLAB Function/2(T) -> Torque [body frame][N m]/1
  MATLAB Function/1(F) -> Force [body frame][N]/1
  Constant/1 -> MATLAB Function/3(Spacecraft)
  Vector rotate/1 -> MATLAB Function/2(relVel)
  Constant1/1 -> Sum/2
  Constant2/1 -> Gain/1
  Gain/1 -> Cross Product/1
  Cross Product/1 -> Sum1/1
  S/c velocity [Earth inertial frame][km/s]/1 -> Sum1/2
  Sum1/1 -> Vector rotate/2
  Sum/1 -> Air density/1(Height)
  Air density/1(Air density) -> MATLAB Function/1(rho)
  S/c position [Earth inertial frame][km]/1 -> Vector magnitude and direction1/1, Cross Product/2
  Vector magnitude and direction1/2 -> Terminator/1

== system main/Real physics/BF to IF ==
  Torque [BF][Nm] : Inport
  Constant : Constant  Value=Spacecraft.str.qIB
  Quaternion Rotation1 : aerolibutil/Quaternion Rotation
  Torque [IF][Nm] : Outport
  wires:
  Quaternion Rotation1/1 -> Torque [IF][Nm]/1
  Torque [BF][Nm]/1 -> Quaternion Rotation1/2
  Constant/1 -> Quaternion Rotation1/1

== system main/Real physics/Gravity gradient ==
  q_I/N : Inport
  s/c position [NF][km] : Inport  Port=2
  Constant : Constant  Value=Earth.mu
  Constant1 : Constant  Value=Spacecraft.str.inertia
  MATLAB Function : MATLAB Function  TreatAsAtomicUnit=on
  Quaternion Rotation : aerolibutil/Quaternion Rotation
  Torque [IF][Nm] : Outport
  wires:
  q_I/N/1 -> Quaternion Rotation/1
  s/c position [NF][km]/1 -> Quaternion Rotation/2
  MATLAB Function/1(torque_IF) -> Torque [IF][Nm]/1
  Constant/1 -> MATLAB Function/1(mu)
  Constant1/1 -> MATLAB Function/2(J)
  Quaternion Rotation/1 -> MATLAB Function/3(position_IF)

== system main/Real physics/IF to BF ==
  Angular velocity [IF][rad/s] : Inport
  q_I/N : Inport  Port=2
  Constant : Constant  Value=Spacecraft.str.qIB
  Quaternion Conjugate : aerolibutil/Quaternion Conjugate
      settings: SourceProductBaseCode=AE
  Quaternion Multiplication : aerolibutil/Quaternion Multiplication
  Quaternion Rotation1 : aerolibutil/Quaternion Rotation
  Angular velocity [BF][rad/s] : Outport
  q_B/N : Outport  Port=2
  wires:
  q_I/N/1 -> Quaternion Multiplication/1
  Quaternion Multiplication/1 -> q_B/N/1
  Constant/1 -> Quaternion Conjugate/1
  Quaternion Rotation1/1 -> Angular velocity [BF][rad/s]/1
  Angular velocity [IF][rad/s]/1 -> Quaternion Rotation1/2
  Quaternion Conjugate/1 -> Quaternion Multiplication/2, Quaternion Rotation1/1

== system main/Real physics/Magnetic dipole ==
  q_B/N : Inport
  s/c position [NF][km] : Inport  Port=2
  Constant : Constant  Value=Spacecraft.str.magDip
  Cross Product : vrlib/Utilities/Cross Product
  Subsystem2 : Subsystem
  T [BF] : Outport
  wires:
  Constant/1 -> Cross Product/1
  q_B/N/1 -> Subsystem2/1(q_A/B)
  s/c position [NF][km]/1 -> Subsystem2/2(r_NF)
  Subsystem2/1(B [BF]) -> Cross Product/2
  Cross Product/1 -> T [BF]/1

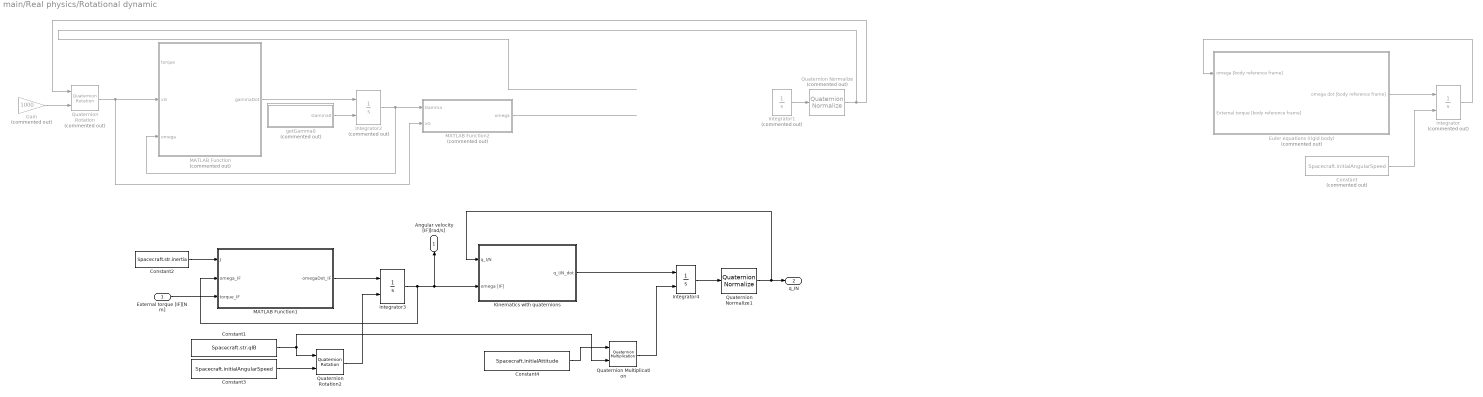
== system main/Real physics/Rotational dynamic ==
  External torque [IF][N m] : Inport
  Constant : Constant  Commented=on  Value=Spacecraft.initialAngularSpeed
  Constant1 : Constant  Value=Spacecraft.str.qIB
  Constant2 : Constant  Value=Spacecraft.str.inertia
  Constant3 : Constant  Value=Spacecraft.initialAngularSpeed
  Constant4 : Constant  Value=Spacecraft.initialAttitude
  "Euler equations (rigid body) " : Subsystem  Commented=on
  Gain : Gain  Commented=on  Gain=1000
  Integrator : Integrator  Commented=on  InitialConditionSource=external  InitialCondition=initCond
  Integrator1 : Integrator  Commented=on  InitialCondition=Spacecraft.initialAttitude
  Integrator2 : Integrator  Commented=on  InitialConditionSource=external  InitialCondition=initCond
  Integrator3 : Integrator  InitialConditionSource=external  InitialCondition=initCond
  Integrator4 : Integrator  InitialConditionSource=external  InitialCondition=Spacecraft.initialAttitude
  Kinematics with quaternions : Subsystem
  MATLAB Function : MATLAB Function  Commented=on  TreatAsAtomicUnit=on
  MATLAB Function1 : MATLAB Function  TreatAsAtomicUnit=on
  MATLAB Function2 : MATLAB Function  Commented=on  TreatAsAtomicUnit=on
  Quaternion Multiplication : aerolibutil/Quaternion Multiplication
  Quaternion Normalize : sharedutil/Quaternion Normalize  Commented=on  aMode=aMode
      settings: SourceProductBaseCode=AE,PW,DR,MT,UV,VE
  Quaternion Normalize1 : sharedutil/Quaternion Normalize  aMode=aMode
      settings: SourceProductBaseCode=AE,PW,DR,MT,UV,VE
  Quaternion Rotation : aerolibutil/Quaternion Rotation  Commented=on
  Quaternion Rotation2 : aerolibutil/Quaternion Rotation
  getGamma0 : Subsystem  Commented=on
  Angular velocity [IF][rad/s] : Outport  OutDataTypeStr=double  Unit=rad/s  PortDimensions=3
  q_IN : Outport  Port=2  OutDataTypeStr=double  Unit=1  PortDimensions=4
  wires:
  ? -> ?
  Constant/1 -> Integrator/2
  Integrator/1 -> "Euler equations (rigid body) "/1(omega [body reference frame])
  "Euler equations (rigid body) "/1(omega dot [body reference frame]) -> Integrator/1
  ? -> Integrator1/1
  Integrator1/1 -> Quaternion Normalize/1
  Quaternion Normalize/1 -> Quaternion Rotation/1
  Gain/1 -> Quaternion Rotation/2
  MATLAB Function/1(gammaDot) -> Integrator2/1
  Integrator2/1 -> MATLAB Function2/1(Gamma), MATLAB Function/3(omega)
  Quaternion Rotation/1 -> MATLAB Function2/2(vG), MATLAB Function/2(vG)
  MATLAB Function2/1(omega) -> ?
  getGamma0/1(Gamma0) -> Integrator2/2
  MATLAB Function1/1(omegaDot_IF) -> Integrator3/1
  Integrator4/1 -> Quaternion Normalize1/1
  Kinematics with quaternions/1(q_I/N_dot) -> Integrator4/1
  Quaternion Normalize1/1 -> Kinematics with quaternions/1(q_I/N), q_IN/1
  External torque [IF][N m]/1 -> MATLAB Function1/3(torque_IF)
  Quaternion Rotation2/1 -> Integrator3/2
  Constant3/1 -> Quaternion Rotation2/2
  Integrator3/1 -> MATLAB Function1/2(omega_IF), Kinematics with quaternions/2(omega [IF]), Angular velocity [IF][rad/s]/1
  Constant4/1 -> Quaternion Multiplication/1
  Constant1/1 -> Quaternion Multiplication/2, Quaternion Rotation2/1
  Quaternion Multiplication/1 -> Integrator4/2
  Constant2/1 -> MATLAB Function1/1(J)

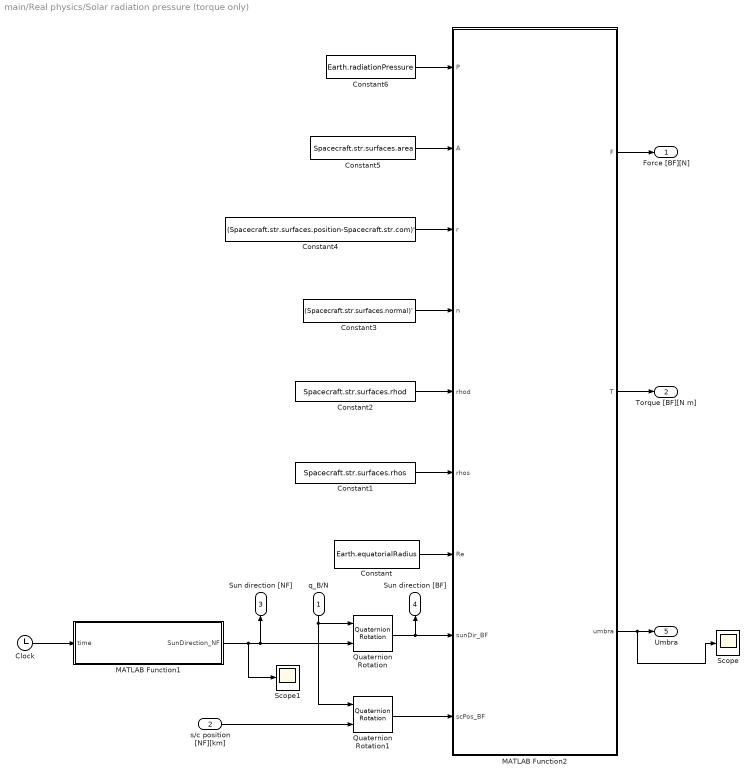
== system main/Real physics/Solar radiation pressure (torque only) ==
  q_B/N : Inport
  s/c position [NF][km] : Inport  Port=2
  Clock : Clock
  Constant : Constant  Value=Earth.equatorialRadius
  Constant1 : Constant  Value=Spacecraft.str.surfaces.rhos
  Constant2 : Constant  Value=Spacecraft.str.surfaces.rhod
  Constant3 : Constant  Value=(Spacecraft.str.surfaces.normal)'
  Constant4 : Constant  Value=(Spacecraft.str.surfaces.position-Spacecraft.str.com)'
  Constant5 : Constant  Value=Spacecraft.str.surfaces.area
  Constant6 : Constant  Value=Earth.radiationPressure
  MATLAB Function1 : MATLAB Function  TreatAsAtomicUnit=on
  MATLAB Function2 : MATLAB Function  TreatAsAtomicUnit=on
  Quaternion Rotation : aerolibutil/Quaternion Rotation
  Quaternion Rotation1 : aerolibutil/Quaternion Rotation
  Scope : Scope
  Scope1 : Scope
  Force [BF][N] : Outport  OutDataTypeStr=double  Unit=N
  Torque [BF][N m] : Outport  Port=2  OutDataTypeStr=double  Unit=N*m
  Sun direction [NF] : Outport  Port=3
  Sun direction [BF] : Outport  Port=4
  Umbra : Outport  Port=5
  wires:
  Clock/1 -> MATLAB Function1/1(time)
  MATLAB Function1/1(SunDirection_NF) -> Scope1/1, Quaternion Rotation/2, Sun direction [NF]/1
  q_B/N/1 -> Quaternion Rotation/1, Quaternion Rotation1/1
  Quaternion Rotation/1 -> MATLAB Function2/8(sunDir_BF), Sun direction [BF]/1
  Quaternion Rotation1/1 -> MATLAB Function2/9(scPos_BF)
  s/c position [NF][km]/1 -> Quaternion Rotation1/2
  MATLAB Function2/2(T) -> Torque [BF][N m]/1
  MATLAB Function2/1(F) -> Force [BF][N]/1
  MATLAB Function2/3(umbra) -> Scope/1, Umbra/1
  Constant/1 -> MATLAB Function2/7(Re)
  Constant1/1 -> MATLAB Function2/6(rhos)
  Constant6/1 -> MATLAB Function2/1(P)
  Constant5/1 -> MATLAB Function2/2(A)
  Constant4/1 -> MATLAB Function2/3(r)
  Constant3/1 -> MATLAB Function2/4(n)
  Constant2/1 -> MATLAB Function2/5(rhod)

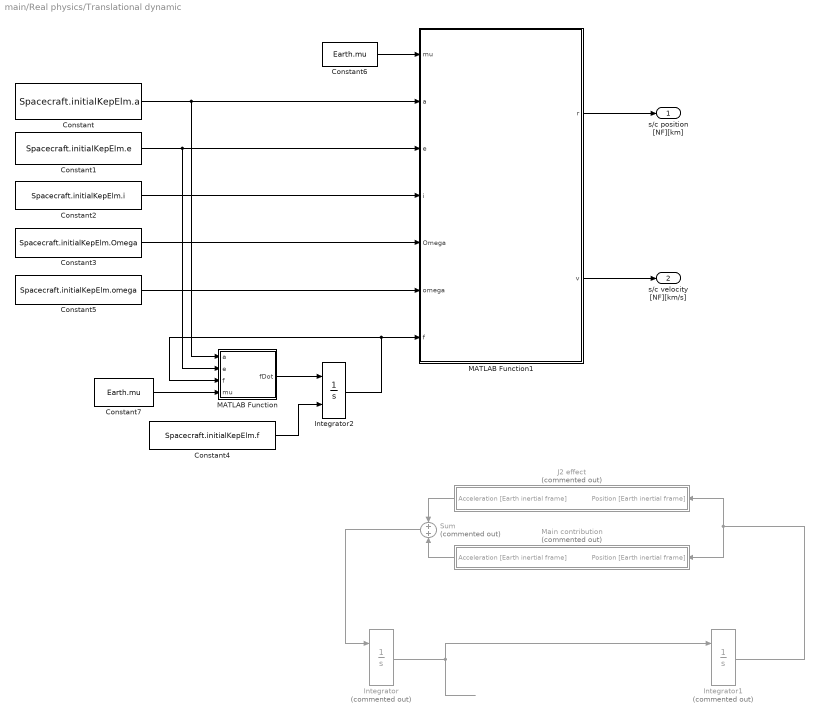
== system main/Real physics/Translational dynamic ==
  Constant : Constant  Value=Spacecraft.initialKepElm.a
  Constant1 : Constant  Value=Spacecraft.initialKepElm.e
  Constant2 : Constant  Value=Spacecraft.initialKepElm.i
  Constant3 : Constant  Value=Spacecraft.initialKepElm.Omega
  Constant4 : Constant  Value=Spacecraft.initialKepElm.f
  Constant5 : Constant  Value=Spacecraft.initialKepElm.omega
  Constant6 : Constant  Value=Earth.mu
  Constant7 : Constant  Value=Earth.mu
  Integrator : Integrator  Commented=on  InitialConditionSource=external  AbsoluteTolerance=1e-14
  Integrator1 : Integrator  Commented=on  InitialConditionSource=external  AbsoluteTolerance=1e-14
  Integrator2 : Integrator  InitialConditionSource=external  AbsoluteTolerance=1e-14
  J2 effect : Subsystem  Commented=on
  MATLAB Function : MATLAB Function  TreatAsAtomicUnit=on
  MATLAB Function1 : MATLAB Function  TreatAsAtomicUnit=on
  Main contribution : Subsystem  Commented=on
  Sum : Sum  Commented=on
  s/c position [NF][km] : Outport
  s/c velocity [NF][km/s] : Outport  Port=2
  wires:
  ? -> Integrator1/2
  Integrator/1 -> Integrator1/1
  Integrator1/1 -> Main contribution/1(Position [Earth inertial frame]), J2 effect/1(Position [Earth inertial frame])
  J2 effect/1(Acceleration [Earth inertial frame]) -> Sum/1
  Main contribution/1(Acceleration [Earth inertial frame]) -> Sum/2
  Sum/1 -> Integrator/1
  Constant4/1 -> Integrator2/2
  Constant5/1 -> MATLAB Function1/6(omega)
  Constant3/1 -> MATLAB Function1/5(Omega)
  Constant2/1 -> MATLAB Function1/4(i)
  Constant1/1 -> MATLAB Function1/3(e), MATLAB Function/2(e)
  Constant/1 -> MATLAB Function1/2(a), MATLAB Function/1(a)
  MATLAB Function1/1(r) -> s/c position [NF][km]/1
  MATLAB Function1/2(v) -> s/c velocity [NF][km/s]/1
  Constant6/1 -> MATLAB Function1/1(mu)
  Constant7/1 -> MATLAB Function/4(mu)
  MATLAB Function/1(fDot) -> Integrator2/1
  Integrator2/1 -> MATLAB Function/3(f), MATLAB Function1/7(f)

== system main/Solve Whabba's problem/Angles 2 vector ==
  In1 : Inport
  Constant : Constant
  Demux : Demux  Outputs=2
  Demux1 : Demux  Outputs=3
  Divide : Product  Inputs=/*
  Mux : Mux  Inputs=3
  Sqrt : Sqrt  SaturateOnIntegerOverflow=on
  Square : Math  Operator=square  SaturateOnIntegerOverflow=on
  Sum : Sum  Inputs=+++
  Tan : Trigonometry  Operator=tan
  Out1 : Outport
  wires:
  Divide/1 -> Out1/1
  Square/1 -> Demux1/1
  Demux1/3 -> Sum/3
  Sum/1 -> Sqrt/1
  Demux/2 -> Mux/2
  Mux/1 -> Divide/2, Square/1
  Demux1/2 -> Sum/2
  In1/1 -> Tan/1
  Demux/1 -> Mux/1
  Sqrt/1 -> Divide/1
  Constant/1 -> Mux/3
  Tan/1 -> Demux/1
  Demux1/1 -> Sum/1

== system main/Solve Whabba's problem/Angles 2 vector1 ==
  Star 2 : Inport
  Constant : Constant
  Demux : Demux  Outputs=2
  Demux1 : Demux  Outputs=3
  Divide : Product  Inputs=/*
  Mux : Mux  Inputs=3
  Sqrt : Sqrt  SaturateOnIntegerOverflow=on
  Square : Math  Operator=square  SaturateOnIntegerOverflow=on
  Sum : Sum  Inputs=+++
  Tan : Trigonometry  Operator=tan
  Out1 : Outport
  wires:
  Divide/1 -> Out1/1
  Square/1 -> Demux1/1
  Demux1/3 -> Sum/3
  Sum/1 -> Sqrt/1
  Demux/2 -> Mux/2
  Mux/1 -> Divide/2, Square/1
  Demux1/2 -> Sum/2
  Star 2/1 -> Tan/1
  Demux/1 -> Mux/1
  Sqrt/1 -> Divide/1
  Constant/1 -> Mux/3
  Tan/1 -> Demux/1
  Demux1/1 -> Sum/1

== system main/Solve Whabba's problem/Angles 2 vector2 ==
  Star 3 : Inport
  Constant : Constant
  Demux : Demux  Outputs=2
  Demux1 : Demux  Outputs=3
  Divide : Product  Inputs=/*
  Mux : Mux  Inputs=3
  Sqrt : Sqrt  SaturateOnIntegerOverflow=on
  Square : Math  Operator=square  SaturateOnIntegerOverflow=on
  Sum : Sum  Inputs=+++
  Tan : Trigonometry  Operator=tan
  Out1 : Outport
  wires:
  Divide/1 -> Out1/1
  Square/1 -> Demux1/1
  Demux1/3 -> Sum/3
  Sum/1 -> Sqrt/1
  Demux/2 -> Mux/2
  Mux/1 -> Divide/2, Square/1
  Demux1/2 -> Sum/2
  Star 3/1 -> Tan/1
  Demux/1 -> Mux/1
  Sqrt/1 -> Divide/1
  Constant/1 -> Mux/3
  Tan/1 -> Demux/1
  Demux1/1 -> Sum/1

== system main/Star sensor/Vector 2 angles ==
  vec : Inport
  Atan1 : Trigonometry  Operator=atan2
  Atan2 : Trigonometry  Operator=atan2
  Demux : Demux  Outputs=3
  Mux : Mux  Inputs=2
  Random Source : dspsrcs4/Random Source  Commented=on  SrcType=Gaussian  NormMethod=Ziggurat  CltLength=12  MinVal=0  MaxVal=1  MeanVal=0  VarVal=Sensors.starTracker.acc  RepMode=Not repeatable  rawSeed=1  IsInherit=off  SampMode=Discrete  SampTime=1/Sensors.starTracker.freq  SampFrame=2  DataType=Double  OutComplex=Real  OutputFrames=off
  Subsystem : Subsystem
  Star 1 : Outport
  wires:
  Mux/1 -> Star 1/1
  Atan1/1 -> Mux/2
  Demux/3 -> Atan2/2, Atan1/2
  Atan2/1 -> Mux/1
  Demux/2 -> Atan1/1
  Demux/1 -> Atan2/1
  vec/1 -> Subsystem/1(vec)
  Subsystem/1(vec_rot) -> Demux/1

== system main/Star sensor/Vector 2 angles1 ==
  vec : Inport
  Atan1 : Trigonometry  Operator=atan2
  Atan2 : Trigonometry  Operator=atan2
  Demux : Demux  Outputs=3
  Mux : Mux  Inputs=2
  Random Source : dspsrcs4/Random Source  Commented=on  SrcType=Gaussian  NormMethod=Ziggurat  CltLength=12  MinVal=0  MaxVal=1  MeanVal=0  VarVal=Sensors.starTracker.acc  RepMode=Not repeatable  rawSeed=1  IsInherit=off  SampMode=Discrete  SampTime=1/Sensors.starTracker.freq  SampFrame=2  DataType=Double  OutComplex=Real  OutputFrames=off
  Subsystem : Subsystem
  Star 1 : Outport
  wires:
  Mux/1 -> Star 1/1
  Atan1/1 -> Mux/2
  Demux/3 -> Atan2/2, Atan1/2
  Atan2/1 -> Mux/1
  Demux/2 -> Atan1/1
  Demux/1 -> Atan2/1
  vec/1 -> Subsystem/1(vec)
  Subsystem/1(vec_rot) -> Demux/1

== system main/Star sensor/Vector 2 angles2 ==
  vec : Inport
  Atan1 : Trigonometry  Operator=atan2
  Atan2 : Trigonometry  Operator=atan2
  Demux : Demux  Outputs=3
  Mux : Mux  Inputs=2
  Random Source : dspsrcs4/Random Source  Commented=on  SrcType=Gaussian  NormMethod=Ziggurat  CltLength=12  MinVal=0  MaxVal=1  MeanVal=0  VarVal=Sensors.starTracker.acc  RepMode=Not repeatable  rawSeed=1  IsInherit=off  SampMode=Discrete  SampTime=1/Sensors.starTracker.freq  SampFrame=2  DataType=Double  OutComplex=Real  OutputFrames=off
  Subsystem : Subsystem
  Star 1 : Outport
  wires:
  Mux/1 -> Star 1/1
  Atan1/1 -> Mux/2
  Demux/3 -> Atan2/2, Atan1/2
  Atan2/1 -> Mux/1
  Demux/2 -> Atan1/1
  Demux/1 -> Atan2/1
  vec/1 -> Subsystem/1(vec)
  Subsystem/1(vec_rot) -> Demux/1

== system main/Star sensor/Vector 2 angles3 ==
  vec : Inport
  Atan1 : Trigonometry  Operator=atan2
  Atan2 : Trigonometry  Operator=atan2
  Demux : Demux  Outputs=3
  Mux : Mux  Inputs=2
  Random Source : dspsrcs4/Random Source  Commented=on  SrcType=Gaussian  NormMethod=Ziggurat  CltLength=12  MinVal=0  MaxVal=1  MeanVal=0  VarVal=Sensors.starTracker.acc  RepMode=Not repeatable  rawSeed=1  IsInherit=off  SampMode=Discrete  SampTime=1/Sensors.starTracker.freq  SampFrame=2  DataType=Double  OutComplex=Real  OutputFrames=off
  Subsystem : Subsystem
  Star 1 : Outport
  wires:
  Mux/1 -> Star 1/1
  Atan1/1 -> Mux/2
  Demux/3 -> Atan2/2, Atan1/2
  Atan2/1 -> Mux/1
  Demux/2 -> Atan1/1
  Demux/1 -> Atan2/1
  vec/1 -> Subsystem/1(vec)
  Subsystem/1(vec_rot) -> Demux/1

== system main/State estimator/State 2 attitude and bias ==
  xHat : Inport
  Demux1 : Demux  Outputs=7
  Mux2 : Mux
  Mux3 : Mux  Inputs=3
  Body frame attitude [ECI] : Outport
  Gyro bias [body frame] : Outport  Port=2
  wires:
  Mux2/1 -> Body frame attitude [ECI]/1
  Demux1/2 -> Mux2/2
  Mux3/1 -> Gyro bias [body frame]/1
  Demux1/7 -> Mux3/3
  Demux1/1 -> Mux2/1
  Demux1/3 -> Mux2/3
  Demux1/5 -> Mux3/1
  xHat/1 -> Demux1/1
  Demux1/6 -> Mux3/2
  Demux1/4 -> Mux2/4

== system main/Subsystem1/Sun sensor reading ==
  True Sun position [body reference frame][km] : Inport  OutDataTypeStr=double  Unit=km
  q_S/B : Inport  Port=2
  Atan3 : Trigonometry  Operator=atan2
  Atan4 : Trigonometry  Operator=atan2
  Demux2 : Demux  Outputs=3
  Mux1 : Mux  Inputs=2
  Normalize Vector : vrlib/Utilities/Normalize Vector  maxzero=0
  Quaternion Rotation : aerolibutil/Quaternion Rotation
  Saturation1 : Saturate  UpperLimit=Sensors.sunSensor.fow  LowerLimit=-Sensors.sunSensor.fow
  Subsystem : Subsystem
  Zero-Order Hold : ZeroOrderHold  SampleTime=1/Sensors.sunSensor.freq
  Sun angles position [sensor axis] : Outport  OutDataTypeStr=double  Unit=1
  wires:
  True Sun position [body reference frame][km]/1 -> Zero-Order Hold/1
  q_S/B/1 -> Quaternion Rotation/1
  Zero-Order Hold/1 -> Normalize Vector/1
  Normalize Vector/1 -> Quaternion Rotation/2
  Quaternion Rotation/1 -> Subsystem/1(vec)
  Demux2/3 -> Atan3/2, Atan4/2
  Demux2/1 -> Atan4/1
  Atan4/1 -> Mux1/1
  Atan3/1 -> Mux1/2
  Mux1/1 -> Saturation1/1
  Subsystem/1(vec_rot) -> Demux2/1
  Demux2/2 -> Atan3/1
  Saturation1/1 -> Sun angles position [sensor axis]/1

== system main/Subsystem1/Sun sensor reading1 ==
  True Sun position [body reference frame][km] : Inport  OutDataTypeStr=double  Unit=km
  q_S/B : Inport  Port=2
  Atan3 : Trigonometry  Operator=atan2
  Atan4 : Trigonometry  Operator=atan2
  Demux2 : Demux  Outputs=3
  Mux1 : Mux  Inputs=2
  Normalize Vector : vrlib/Utilities/Normalize Vector  maxzero=0
  Quaternion Rotation : aerolibutil/Quaternion Rotation
  Saturation1 : Saturate  UpperLimit=Sensors.sunSensor.fow  LowerLimit=-Sensors.sunSensor.fow
  Subsystem : Subsystem
  Zero-Order Hold : ZeroOrderHold  SampleTime=1/Sensors.sunSensor.freq
  Sun angles position [sensor axis] : Outport  OutDataTypeStr=double  Unit=1
  wires:
  True Sun position [body reference frame][km]/1 -> Zero-Order Hold/1
  q_S/B/1 -> Quaternion Rotation/1
  Zero-Order Hold/1 -> Normalize Vector/1
  Normalize Vector/1 -> Quaternion Rotation/2
  Quaternion Rotation/1 -> Subsystem/1(vec)
  Demux2/3 -> Atan3/2, Atan4/2
  Demux2/1 -> Atan4/1
  Atan4/1 -> Mux1/1
  Atan3/1 -> Mux1/2
  Mux1/1 -> Saturation1/1
  Subsystem/1(vec_rot) -> Demux2/1
  Demux2/2 -> Atan3/1
  Saturation1/1 -> Sun angles position [sensor axis]/1

== system main/Subsystem1/Sun sensor reading2 ==
  True Sun position [body reference frame][km] : Inport  OutDataTypeStr=double  Unit=km
  q_S/B : Inport  Port=2
  Atan3 : Trigonometry  Operator=atan2
  Atan4 : Trigonometry  Operator=atan2
  Demux2 : Demux  Outputs=3
  Mux1 : Mux  Inputs=2
  Normalize Vector : vrlib/Utilities/Normalize Vector  maxzero=0
  Quaternion Rotation : aerolibutil/Quaternion Rotation
  Saturation1 : Saturate  UpperLimit=Sensors.sunSensor.fow  LowerLimit=-Sensors.sunSensor.fow
  Subsystem : Subsystem
  Zero-Order Hold : ZeroOrderHold  SampleTime=1/Sensors.sunSensor.freq
  Sun angles position [sensor axis] : Outport  OutDataTypeStr=double  Unit=1
  wires:
  True Sun position [body reference frame][km]/1 -> Zero-Order Hold/1
  q_S/B/1 -> Quaternion Rotation/1
  Zero-Order Hold/1 -> Normalize Vector/1
  Normalize Vector/1 -> Quaternion Rotation/2
  Quaternion Rotation/1 -> Subsystem/1(vec)
  Demux2/3 -> Atan3/2, Atan4/2
  Demux2/1 -> Atan4/1
  Atan4/1 -> Mux1/1
  Atan3/1 -> Mux1/2
  Mux1/1 -> Saturation1/1
  Subsystem/1(vec_rot) -> Demux2/1
  Demux2/2 -> Atan3/1
  Saturation1/1 -> Sun angles position [sensor axis]/1
